simulink model "controle_atitude_lqr2"  (R2021b)
settings: Solver=ode45  StartTime=0.0  StopTime=100  MaxStep=0.4  RelTol=1e-3
values from neighbouring files (symbols this model uses):
  b = 5.16e-06    [parametros2.mat]    (also in parametros3.mat = 0.1; parametros4.mat)
  J = [0.00216966666667  0  0; 0  0.00216966666667  0; 0  0  0.00216966666667]    [parametros2.mat]    (also in parametros3.mat)
  Jr = 3e-06    [parametros2.mat]    (also in parametros4.mat = 9.756e-06)
  K4_lqr = [0.162305258799 0.031097907508 -0.386751961034 -0.0999999697508]    [parametros2.mat]
  Kiw = 0.0467    [parametros2.mat]
  Km = 0.0264    [parametros2.mat]
  Kpw = 0.1772    [parametros2.mat]
libraries: aerolibutil x3, sharedutil x3, sharedtransform x2
settings Model: Creator=JRRL  LastModifiedBy=JRRL

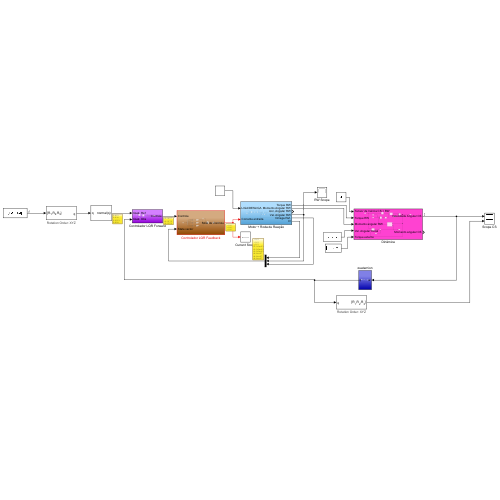
[thumbnail: Simulink's stored preview of the top-level diagram]
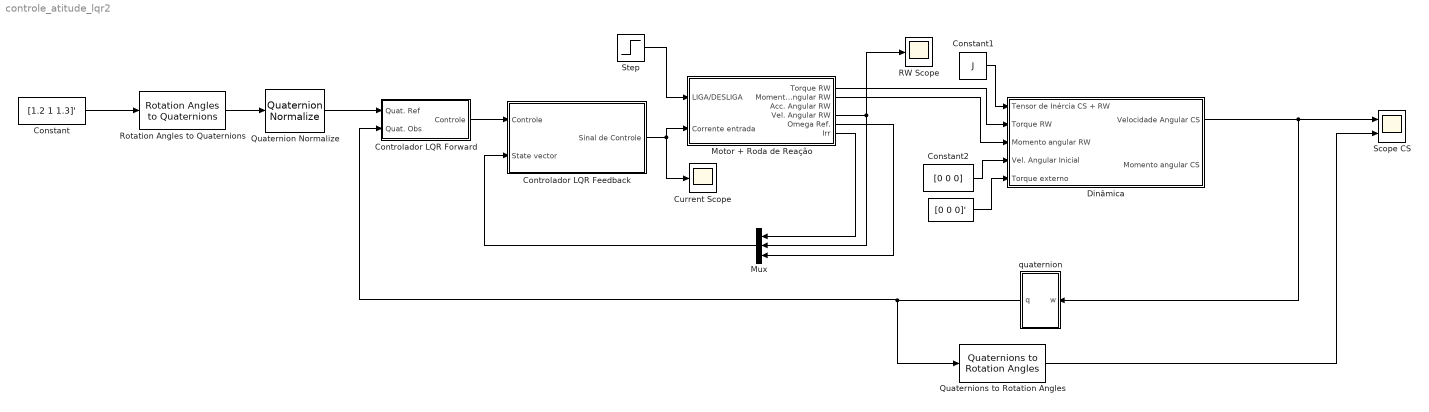
== system controle_atitude_lqr2 ==
  " " : Constant  Value=[0 0 0]'
  Constant : Constant  Value=[1.2 1 1.3]'
  Constant1 : Constant  Value=J
  Constant2 : Constant  Value=[0 0 0]
  Controlador LQR Feedback : Subsystem
  Controlador LQR Forward : Subsystem
  Current Scope : Scope
  Dinâmica : Subsystem
  Motor + Roda de Reação : Subsystem
  Mux : Mux  Inputs=3
  Quaternion Normalize : sharedutil/Quaternion Normalize  aMode=aMode
      settings: SourceProductBaseCode=AE,PW,DR,MT,UV,VE
  Quaternions to Rotation Angles : sharedtransform/Quaternions to Rotation Angles  rotationOrder=XYZ  aMode=aMode
      settings: SourceProductBaseCode=AE,PW,DR,MT,UV,VE
  RW Scope : Scope
  Rotation Angles to Quaternions : sharedtransform/Rotation Angles to Quaternions  rotationOrder=XYZ  aMode=aMode
      settings: SourceProductBaseCode=AE,PW,DR,MT,UV,VE
  Scope CS : Scope  NumInputPorts=2
  Step : Step  Time=100  Before=1  SampleTime=0
  quaternion : Subsystem
  wires:
  Constant1/1 -> Dinâmica/1(Tensor de Inércia CS + RW)
  Dinâmica/1(Velocidade Angular CS) -> Scope CS/1, quaternion/1(w)
  Constant2/1 -> Dinâmica/4(Vel. Angular Inicial)
  " "/1 -> Dinâmica/5(Torque externo)
  quaternion/1(q) -> Controlador LQR Forward/2(Quat. Obs), Quaternions to Rotation Angles/1
  Constant/1 -> Rotation Angles to Quaternions/1
  Rotation Angles to Quaternions/1 -> Quaternion Normalize/1
  Quaternions to Rotation Angles/1 -> Scope CS/2
  Quaternion Normalize/1 -> Controlador LQR Forward/1(Quat. Ref)
  Step/1 -> Motor + Roda de Reação/1(LIGA/DESLIGA)
  Motor + Roda de Reação/1(Torque RW) -> Dinâmica/2(Torque RW)
  Motor + Roda de Reação/2(Momento Angular RW) -> Dinâmica/3(Momento angular RW)
  Motor + Roda de Reação/4(Vel. Angular RW) -> Mux/2, RW Scope/1
  Motor + Roda de Reação/6(Irr) -> Mux/1
  Motor + Roda de Reação/5(Omega Ref.) -> Mux/3
  Controlador LQR Feedback/1(Sinal de Controle) -> Motor + Roda de Reação/2(Corrente entrada), Current Scope/1
  Mux/1 -> Controlador LQR Feedback/2(State vector)
  Controlador LQR Forward/1(Controle) -> Controlador LQR Feedback/1(Controle)

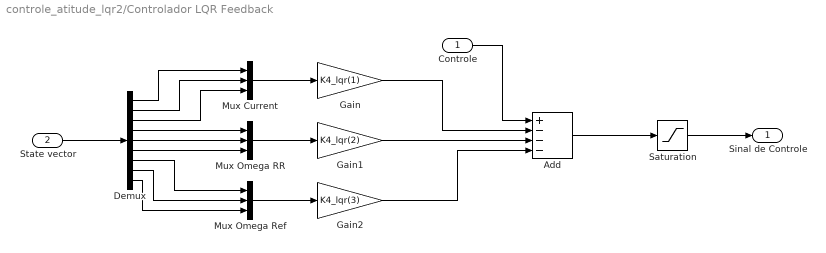
== system controle_atitude_lqr2/Controlador LQR Feedback ==
  Controle : Inport
  State vector : Inport  Port=2
  Add : Sum  Inputs=+---
  Demux : Demux  Outputs=9
  Gain : Gain  Gain=K4_lqr(1)
  Gain1 : Gain  Gain=K4_lqr(2)
  Gain2 : Gain  Gain=K4_lqr(3)
  Mux Current : Mux  Inputs=3
  Mux Omega RR : Mux  Inputs=3
  Mux Omega Ref : Mux  Inputs=3
  Saturation : Saturate  UpperLimit=100  LowerLimit=-100
  Sinal de Controle : Outport
  wires:
  State vector/1 -> Demux/1
  Demux/1 -> Mux Current/1
  Demux/2 -> Mux Current/2
  Demux/3 -> Mux Current/3
  Demux/4 -> Mux Omega RR/1
  Demux/5 -> Mux Omega RR/2
  Demux/6 -> Mux Omega RR/3
  Demux/7 -> Mux Omega Ref/1
  Demux/8 -> Mux Omega Ref/2
  Demux/9 -> Mux Omega Ref/3
  Mux Omega RR/1 -> Gain1/1
  Mux Current/1 -> Gain/1
  Mux Omega Ref/1 -> Gain2/1
  Controle/1 -> Add/1
  Gain/1 -> Add/2
  Gain1/1 -> Add/3
  Gain2/1 -> Add/4
  Add/1 -> Saturation/1
  Saturation/1 -> Sinal de Controle/1

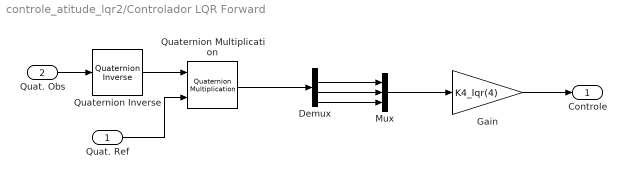
== system controle_atitude_lqr2/Controlador LQR Forward ==
  Quat. Ref : Inport
  Quat. Obs : Inport  Port=2
  Demux : Demux
  Gain : Gain  Gain=K4_lqr(4)
  Mux : Mux  Inputs=3
  Quaternion Inverse : aerolibutil/Quaternion Inverse
  Quaternion Multiplication : aerolibutil/Quaternion Multiplication
  Controle : Outport
  wires:
  Quat. Ref/1 -> Quaternion Multiplication/2
  Quat. Obs/1 -> Quaternion Inverse/1
  Quaternion Inverse/1 -> Quaternion Multiplication/1
  Quaternion Multiplication/1 -> Demux/1
  Demux/3 -> Mux/2
  Demux/2 -> Mux/1
  Demux/4 -> Mux/3
  Mux/1 -> Gain/1
  Gain/1 -> Controle/1

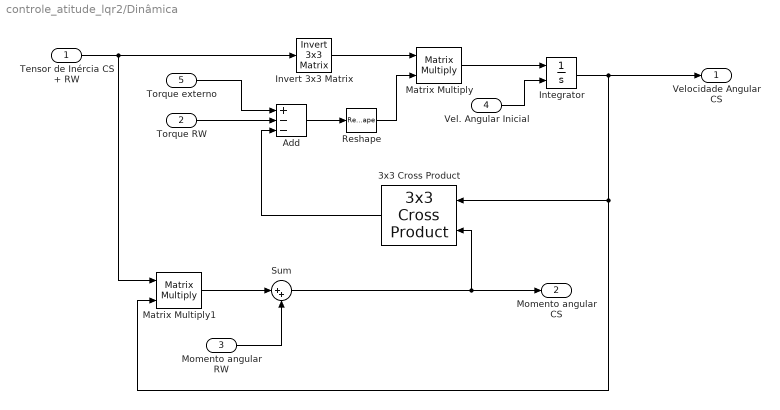
== system controle_atitude_lqr2/Dinâmica ==
  Tensor de Inércia CS + RW : Inport
  Torque RW : Inport  Port=2
  Momento angular RW : Inport  Port=3
  Vel. Angular Inicial : Inport  Port=4
  Torque externo : Inport  Port=5
  3x3 Cross Product : sharedutil/3x3 Cross Product  aMode=aMode
      settings: SourceProductBaseCode=AE,PW,DR,MT,UV,VE
  Add : Sum  Inputs=+--
  Integrator : Integrator  InitialConditionSource=external
  Invert 3x3 Matrix : aerolibutil/Invert  3x3 Matrix
  Matrix Multiply : Product  Multiplication=Matrix(*)
  Matrix Multiply1 : Product  Multiplication=Matrix(*)
  Reshape : Reshape  OutputDimensionality=Column vector (2-D)
  Sum : Sum  Inputs=|++
  Velocidade Angular CS : Outport
  Momento angular CS : Outport  Port=2
  wires:
  Sum/1 -> Momento angular CS/1, 3x3 Cross Product/2
  3x3 Cross Product/1 -> Add/3
  Invert 3x3 Matrix/1 -> Matrix Multiply/1
  Integrator/1 -> Velocidade Angular CS/1, Matrix Multiply1/2, 3x3 Cross Product/1
  Matrix Multiply/1 -> Integrator/1
  Momento angular RW/1 -> Sum/2
  Torque RW/1 -> Add/2
  Tensor de Inércia CS + RW/1 -> Matrix Multiply1/1, Invert 3x3 Matrix/1
  Torque externo/1 -> Add/1
  Vel. Angular Inicial/1 -> Integrator/2
  Add/1 -> Reshape/1
  Matrix Multiply1/1 -> Sum/1
  Reshape/1 -> Matrix Multiply/2

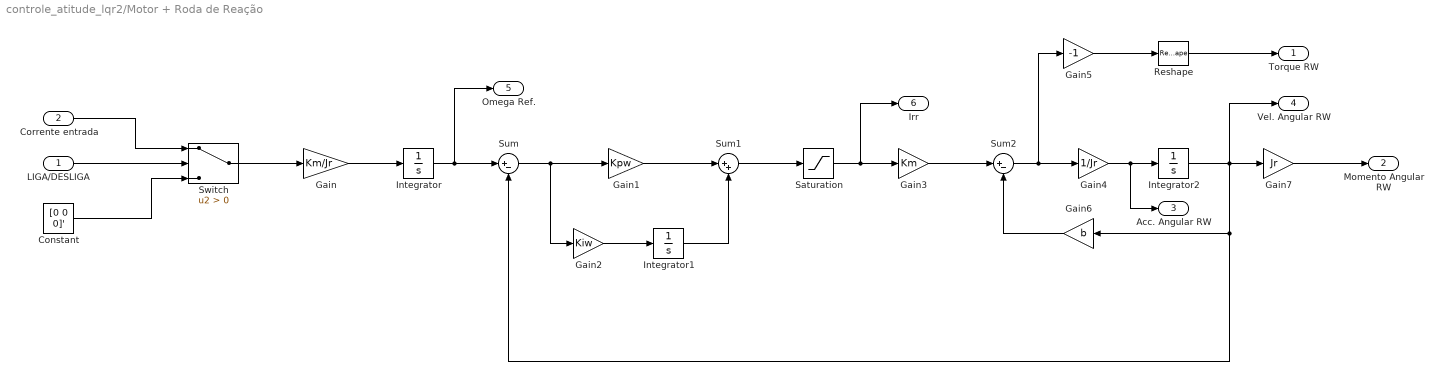
== system controle_atitude_lqr2/Motor + Roda de Reação ==
  LIGA/DESLIGA : Inport
  Corrente entrada : Inport  Port=2
  Constant : Constant  Value=[0 0 0]'
  Gain : Gain  Gain=Km/Jr
  Gain1 : Gain  Gain=Kpw
  Gain2 : Gain  Gain=Kiw
  Gain3 : Gain  Gain=Km
  Gain4 : Gain  Gain=1/Jr
  Gain5 : Gain  Gain=-1
  Gain6 : Gain  Gain=b
  Gain7 : Gain  Gain=Jr
  Integrator : Integrator
  Integrator1 : Integrator
  Integrator2 : Integrator
  Reshape : Reshape  OutputDimensionality=Column vector (2-D)
  Saturation : Saturate
  Sum : Sum  Inputs=|+-
  Sum1 : Sum  Inputs=|++
  Sum2 : Sum  Inputs=|+-
  Switch : Switch  Criteria=u2 > Threshold
  Torque RW : Outport
  Momento Angular RW : Outport  Port=2
  Acc. Angular RW : Outport  Port=3
  Vel. Angular RW : Outport  Port=4
  Omega Ref. : Outport  Port=5
  Irr : Outport  Port=6
  wires:
  Saturation/1 -> Irr/1, Gain3/1
  Gain1/1 -> Sum1/1
  Sum/1 -> Gain2/1, Gain1/1
  Reshape/1 -> Torque RW/1
  Sum1/1 -> Saturation/1
  Gain2/1 -> Integrator1/1
  Sum2/1 -> Gain5/1, Gain4/1
  Integrator2/1 -> Vel. Angular RW/1, Sum/2, Gain6/1, Gain7/1
  Gain4/1 -> Acc. Angular RW/1, Integrator2/1
  Gain7/1 -> Momento Angular RW/1
  Gain6/1 -> Sum2/2
  Gain5/1 -> Reshape/1
  Integrator1/1 -> Sum1/2
  Gain3/1 -> Sum2/1
  Integrator/1 -> Omega Ref./1, Sum/1
  Gain/1 -> Integrator/1
  LIGA/DESLIGA/1 -> Switch/2
  Corrente entrada/1 -> Switch/1
  Constant/1 -> Switch/3
  Switch/1 -> Gain/1

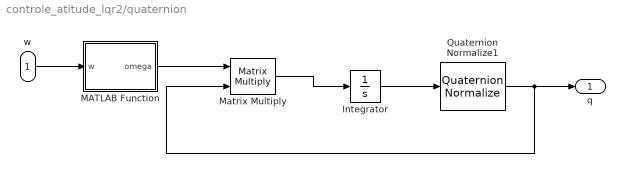
== system controle_atitude_lqr2/quaternion ==
  w : Inport
  Integrator : Integrator  InitialCondition=[1 0 0 0]
  MATLAB Function : MATLAB Function  TreatAsAtomicUnit=on
  Matrix Multiply : Product  Multiplication=Matrix(*)
  Quaternion Normalize1 : sharedutil/Quaternion Normalize  aMode=aMode
      settings: SourceProductBaseCode=AE,PW,DR,MT,UV,VE
  q : Outport
  wires:
  w/1 -> MATLAB Function/1(w)
  MATLAB Function/1(omega) -> Matrix Multiply/1
  Quaternion Normalize1/1 -> q/1, Matrix Multiply/2
  Matrix Multiply/1 -> Integrator/1
  Integrator/1 -> Quaternion Normalize1/1

== matlab function controle_atitude_lqr2/quaternion/MATLAB Function ==
  data: w input; omega output
function omega = fcn(w)
    wx = w(1);
    wy = w(2);
    wz = w(3);
    res = [0 -wx -wy -wz;wx 0 wz -wy;wy -wz 0 wx;wz wy -wx 0];
omega = res;
